simulink model "DCmotor_OL_Ctrl"  (R2022b)
settings: Solver=ode4  StartTime=0.0  StopTime=inf  FixedStep=0.001  RelTol=1e-3  EnableMultiTasking=on
libraries: arduinolib x5, arduinosensorlib x2
settings Model: ExtModeTrigDuration=2  Creator=user  LastModifiedBy=user
settings DataIOCC: ReturnWorkspaceOutputs=off
settings OptimizationCC: EnhancedBackFolding=on  PassReuseOutputArgsAs=Individual arguments  ZeroExternalMemoryAtStartup=off  ZeroInternalMemoryAtStartup=off  MaxStackSize=64  OptimizeBlockOrder=speed  DifferentSizesBufferReuse=on  OptimizationCustomize=off  EfficientTunableParamExpr=on
settings DebuggingCC: ParameterTunabilityLossMsg=error  UnconnectedInputMsg=warning  UnconnectedOutputMsg=warning  UnconnectedLineMsg=warning
settings HardwareCC: ProdBitPerInt=16  ProdBitPerPointer=16  ProdBitPerSizeT=16  ProdBitPerPtrDiffT=16  ProdLargestAtomicFloat=None  ProdWordSize=8  ProdHWDeviceType=Atmel->AVR
settings ModelReferenceCC: EnableRefExpFcnMdlSchedulingChecks=on
settings SFSimCC: MATLABDynamicMemAlloc=off
settings RTWCC: Description=Embedded Coder  SystemTargetFile=ert.tlc  HardwareBoard=Arduino Mega 2560  TLCOptions=-aInlineSetEventsForThisBaseRateFcn=TLC_FALSE -aSuppressMultiTaskScheduler=TLC_FALSE -aRateBasedStepFcn=1  TemplateMakefile=ert_default_tmf  Toolchain=Arduino AVR  BuildConfiguration=Faster Runs  DLArmComputeVersion=19.05
settings CodeAppCC: ForceParamTrailComments=on  IgnoreCustomStorageClasses=off  OperatorAnnotations=on  SimulinkDataObjDesc=on  SFDataObjDesc=on  InsertBlockDesc=on
settings ERTTargetCC: SupportContinuousTime=on  SupportVariableSizeSignals=on  ExtModeTransport=3  ExtModeStaticAlloc=on  ExtModeStaticAllocSize=2048  ExtModeMexFile=ext_xcp  ExtModeIntrfLevel=Level2 - Open

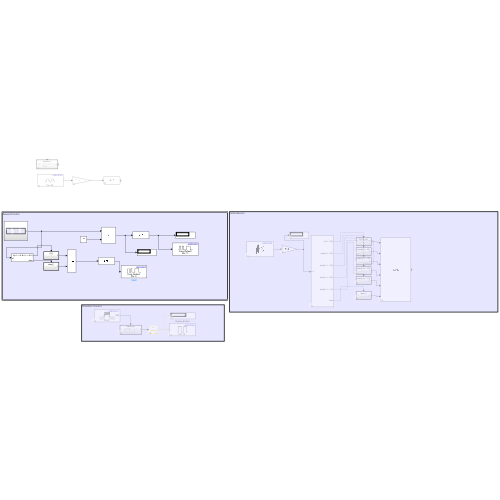
[thumbnail: Simulink's stored preview of the top-level diagram]
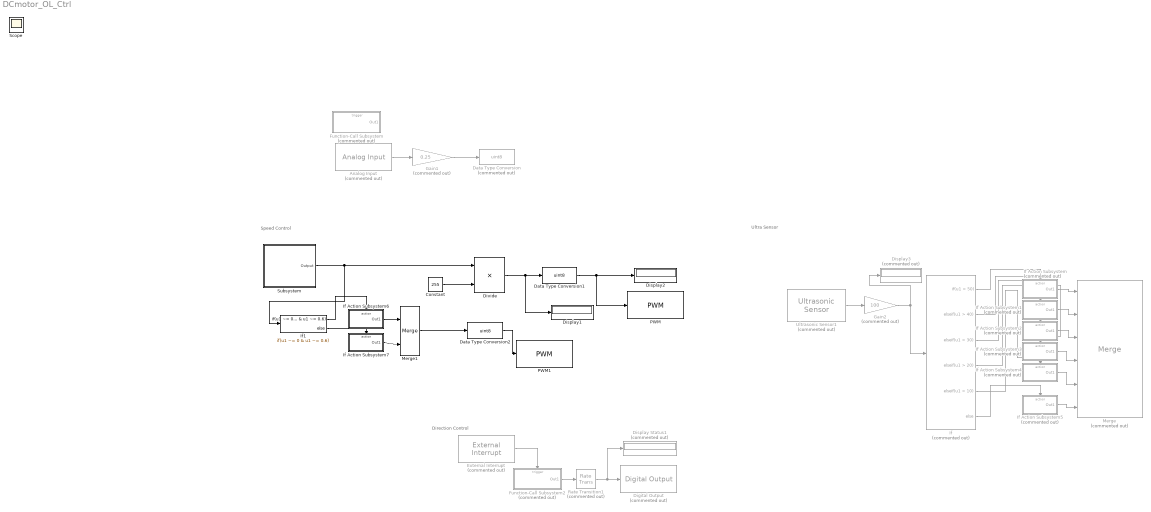
== system DCmotor_OL_Ctrl ==
  note: Speed Control
  note: Ultra Sensor
  note: Direction Control
  Analog Input : arduinolib/Analog Input  Commented=on  pinNumber=0  ReadResultsOnly=off  ConversionTriggerSource=Software  ExternalTriggerType=uint32( 0 )  OutputDataType=uint16  EnableConversionCompleteNotify=off  EnableOuputStatus=off  SampleTime=-1  blockPlatform=arduino
  Constant : Constant  Value=255
  Data Type Conversion : DataTypeConversion  Commented=on  OutDataTypeStr=uint8  SaturateOnIntegerOverflow=off  RndMeth=Floor
  Data Type Conversion1 : DataTypeConversion  OutDataTypeStr=uint8  SaturateOnIntegerOverflow=off  RndMeth=Floor
  Data Type Conversion2 : DataTypeConversion  OutDataTypeStr=uint8  SaturateOnIntegerOverflow=off  RndMeth=Floor
  Digital Output : arduinolib/Digital Output  Commented=on  pinNumber=13  Direction=output  blockPlatform=arduino
  Display Status1 : Display  Commented=on
  Display1 : Display
  Display2 : Display
  Display3 : Display  Commented=on
  Divide : Product  Inputs=**
  External Interrupt : arduinolib/External Interrupt  Commented=on  Pin=2  PullUp=off  Mode=FALLING  InterruptSimulationInput=off
  Function-Call Subsystem : Subsystem  Commented=on  TreatAsAtomicUnit=on
  Function-Call Subsystem2 : Subsystem  Commented=on  TreatAsAtomicUnit=on
  Gain1 : Gain  Commented=on  Gain=0.25
  Gain2 : Gain  Commented=on  Gain=100
  If : If  Commented=on  IfExpression=u1 > 50  ElseIfExpressions=u1 > 40, u1 > 30, u1 > 20, u1 > 10
  If Action Subsystem : Subsystem  Commented=on  TreatAsAtomicUnit=on
  If Action Subsystem1 : Subsystem  Commented=on  TreatAsAtomicUnit=on
  If Action Subsystem2 : Subsystem  Commented=on  TreatAsAtomicUnit=on
  If Action Subsystem3 : Subsystem  Commented=on  TreatAsAtomicUnit=on
  If Action Subsystem4 : Subsystem  Commented=on  TreatAsAtomicUnit=on
  If Action Subsystem5 : Subsystem  Commented=on  TreatAsAtomicUnit=on
  If Action Subsystem6 : Subsystem  TreatAsAtomicUnit=on
  If Action Subsystem7 : Subsystem  TreatAsAtomicUnit=on
  If1 : If  IfExpression=u1 ~= 0 & u1 ~= 0.6
  Merge : Merge  Commented=on  Inputs=6
  Merge1 : Merge  InitialOutput=[0]
  PWM : arduinolib/PWM  pinNumber=11  frequencyType=Default  desiredFrequency=490.2  achievableFrequency=490.2
  PWM1 : arduinolib/PWM  pinNumber=5  frequencyType=Default  desiredFrequency=490.2  achievableFrequency=490.2
  Rate Transition1 : RateTransition  Commented=on  Deterministic=off
  Subsystem : Subsystem
  Ultrasonic Sensor1 : arduinosensorlib/Ultrasonic Sensor  Commented=on  NumSignalPins=2  TrigPin=50  EchoPin=51  SignalPin=3  SampleTime_=0.1  blockPlatform=ARDUINO
  Scope : Scope
  wires:
  Analog Input/1 -> Gain1/1
  Gain1/1 -> Data Type Conversion/1
  Constant/1 -> Divide/2
  Data Type Conversion1/1 -> PWM/1, Display2/1
  Gain2/1 -> Display3/1, If/1
  Ultrasonic Sensor1/1 -> Gain2/1
  If/2 -> If Action Subsystem1/Action
  If/1 -> If Action Subsystem/Action
  If/3 -> If Action Subsystem2/Action
  If/4 -> If Action Subsystem3/Action
  If/5 -> If Action Subsystem4/Action
  If/6 -> If Action Subsystem5/Action
  If Action Subsystem/1(Out1) -> Merge/1
  If Action Subsystem1/1(Out1) -> Merge/2
  If Action Subsystem2/1(Out1) -> Merge/3
  If Action Subsystem3/1(Out1) -> Merge/4
  If Action Subsystem4/1(Out1) -> Merge/5
  If Action Subsystem5/1(Out1) -> Merge/6
  Divide/1 -> Display1/1, Data Type Conversion1/1
  Function-Call Subsystem2/1(Out1) -> Rate Transition1/1
  Rate Transition1/1 -> Display Status1/1, Digital Output/1
  External Interrupt/1 -> Function-Call Subsystem2/Trigger
  Subsystem/1(Output) -> Divide/1, If1/1
  Data Type Conversion2/1 -> PWM1/1
  If Action Subsystem6/1(Out1) -> Merge1/1
  If Action Subsystem7/1(Out1) -> Merge1/2
  If1/1 -> If Action Subsystem6/Action
  If1/2 -> If Action Subsystem7/Action
  Merge1/1 -> Data Type Conversion2/1

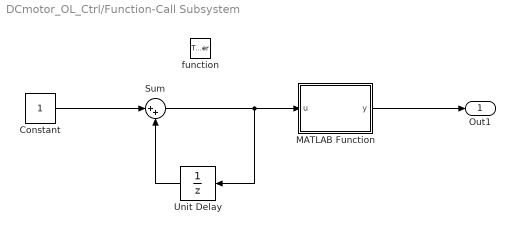
== system DCmotor_OL_Ctrl/Function-Call Subsystem ==
  function : TriggerPort  TriggerType=function-call  VariantControl=(inherit)
  Constant : Constant
  MATLAB Function : MATLAB Function  TreatAsAtomicUnit=on
  Sum : Sum  Inputs=|++
  Unit Delay : UnitDelay  SampleTime=-1  HasFrameUpgradeWarning=on
  Out1 : Outport
  wires:
  Constant/1 -> Sum/1
  Unit Delay/1 -> Sum/2
  Sum/1 -> Unit Delay/1, MATLAB Function/1(u)
  MATLAB Function/1(y) -> Out1/1

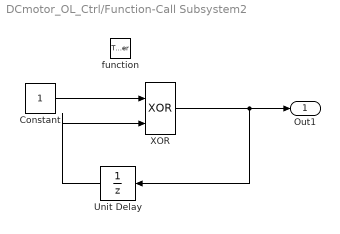
== system DCmotor_OL_Ctrl/Function-Call Subsystem2 ==
  function : TriggerPort  TriggerType=function-call  VariantControl=(inherit)
  Constant : Constant
  Unit Delay : UnitDelay  SampleTime=-1  HasFrameUpgradeWarning=on
  XOR : Logic  Operator=XOR  IconShape=distinctive  AllPortsSameDT=off  OutDataTypeStr=boolean
  Out1 : Outport
  wires:
  Constant/1 -> XOR/1
  Unit Delay/1 -> XOR/2
  XOR/1 -> Unit Delay/1, Out1/1

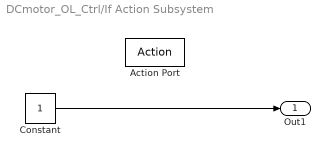
== system DCmotor_OL_Ctrl/If Action Subsystem ==
  Action Port : ActionPort  ActionPortLabel=if(u1 > 50)
  Constant : Constant
  Out1 : Outport
  wires:
  Constant/1 -> Out1/1

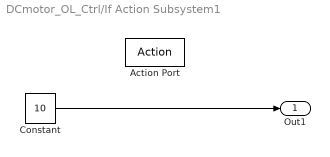
== system DCmotor_OL_Ctrl/If Action Subsystem1 ==
  Action Port : ActionPort  ActionPortLabel=elseif(u1 > 40)
  Constant : Constant  Value=10
  Out1 : Outport
  wires:
  Constant/1 -> Out1/1

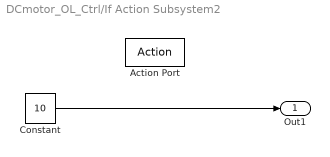
== system DCmotor_OL_Ctrl/If Action Subsystem2 ==
  Action Port : ActionPort  ActionPortLabel=elseif( u1 > 30)
  Constant : Constant  Value=10
  Out1 : Outport
  wires:
  Constant/1 -> Out1/1

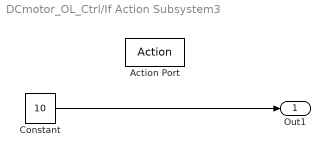
== system DCmotor_OL_Ctrl/If Action Subsystem3 ==
  Action Port : ActionPort  ActionPortLabel=elseif( u1 > 20)
  Constant : Constant  Value=10
  Out1 : Outport
  wires:
  Constant/1 -> Out1/1

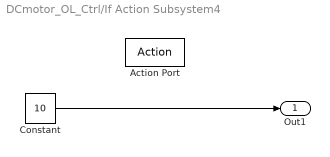
== system DCmotor_OL_Ctrl/If Action Subsystem4 ==
  Action Port : ActionPort  ActionPortLabel=elseif( u1 > 10)
  Constant : Constant  Value=10
  Out1 : Outport
  wires:
  Constant/1 -> Out1/1

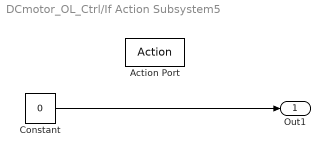
== system DCmotor_OL_Ctrl/If Action Subsystem5 ==
  Action Port : ActionPort  ActionPortLabel=else
  Constant : Constant  Value=0
  Out1 : Outport
  wires:
  Constant/1 -> Out1/1

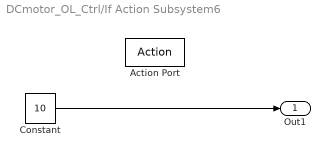
== system DCmotor_OL_Ctrl/If Action Subsystem6 ==
  Action Port : ActionPort  ActionPortLabel=if(u1 ~= 0 & u1 ~= 0.6)
  Constant : Constant  Value=10
  Out1 : Outport
  wires:
  Constant/1 -> Out1/1

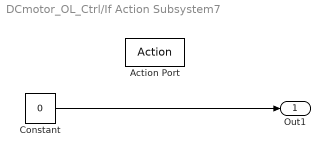
== system DCmotor_OL_Ctrl/If Action Subsystem7 ==
  Action Port : ActionPort  ActionPortLabel=else
  Constant : Constant  Value=0
  Out1 : Outport
  wires:
  Constant/1 -> Out1/1

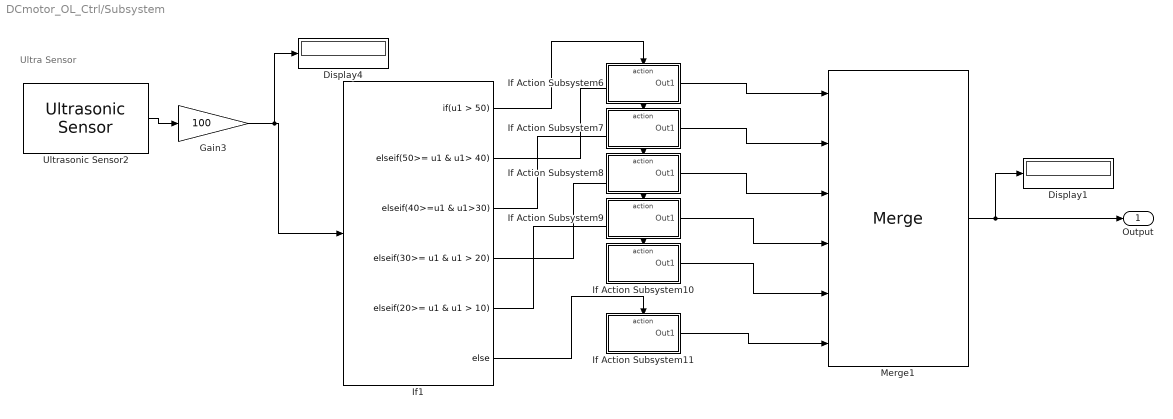
== system DCmotor_OL_Ctrl/Subsystem ==
  note: Ultra Sensor
  Display1 : Display
  Display4 : Display
  Gain3 : Gain  Gain=100
  If Action Subsystem10 : Subsystem  TreatAsAtomicUnit=on
  If Action Subsystem11 : Subsystem  TreatAsAtomicUnit=on
  If Action Subsystem6 : Subsystem  TreatAsAtomicUnit=on
  If Action Subsystem7 : Subsystem  TreatAsAtomicUnit=on
  If Action Subsystem8 : Subsystem  TreatAsAtomicUnit=on
  If Action Subsystem9 : Subsystem  TreatAsAtomicUnit=on
  If1 : If  IfExpression=u1 > 50  ElseIfExpressions=50>= u1 & u1> 40, 40>=u1 & u1>30, 30>= u1 & u1 > 20, 20>= u1 & u1 > 10
  Merge1 : Merge  Inputs=6
  Ultrasonic Sensor2 : arduinosensorlib/Ultrasonic Sensor  NumSignalPins=2  TrigPin=50  EchoPin=51  SignalPin=3  SampleTime_=0.1  blockPlatform=ARDUINO
  Output : Outport
  wires:
  Gain3/1 -> If1/1, Display4/1
  Ultrasonic Sensor2/1 -> Gain3/1
  If Action Subsystem9/1(Out1) -> Merge1/4
  If Action Subsystem11/1(Out1) -> Merge1/6
  If Action Subsystem8/1(Out1) -> Merge1/3
  If Action Subsystem7/1(Out1) -> Merge1/2
  If Action Subsystem6/1(Out1) -> Merge1/1
  If Action Subsystem10/1(Out1) -> Merge1/5
  If1/1 -> If Action Subsystem6/Action
  If1/2 -> If Action Subsystem7/Action
  If1/3 -> If Action Subsystem8/Action
  If1/4 -> If Action Subsystem9/Action
  If1/5 -> If Action Subsystem10/Action
  If1/6 -> If Action Subsystem11/Action
  Merge1/1 -> Display1/1, Output/1

== system DCmotor_OL_Ctrl/Subsystem/If Action Subsystem10 ==
  Action Port : ActionPort  ActionPortLabel=elseif( 20>= u1 & u1 > 10)
  Constant : Constant  Value=0.2
  Out1 : Outport
  wires:
  Constant/1 -> Out1/1

== system DCmotor_OL_Ctrl/Subsystem/If Action Subsystem11 ==
  Action Port : ActionPort  ActionPortLabel=else
  Constant : Constant  Value=0
  Out1 : Outport
  wires:
  Constant/1 -> Out1/1

== system DCmotor_OL_Ctrl/Subsystem/If Action Subsystem6 ==
  Action Port : ActionPort  ActionPortLabel=if(u1 > 50)
  Constant : Constant  Value=0.6
  Out1 : Outport
  wires:
  Constant/1 -> Out1/1

== system DCmotor_OL_Ctrl/Subsystem/If Action Subsystem7 ==
  Action Port : ActionPort  ActionPortLabel=elseif(50>= u1 & u1> 40)
  Constant : Constant  Value=0.5
  Out1 : Outport
  wires:
  Constant/1 -> Out1/1

== system DCmotor_OL_Ctrl/Subsystem/If Action Subsystem8 ==
  Action Port : ActionPort  ActionPortLabel=elseif( 40>=u1 & u1>30)
  Constant : Constant  Value=0.4
  Out1 : Outport
  wires:
  Constant/1 -> Out1/1

== system DCmotor_OL_Ctrl/Subsystem/If Action Subsystem9 ==
  Action Port : ActionPort  ActionPortLabel=elseif( 30>= u1 & u1 > 20)
  Constant : Constant  Value=0.3
  Out1 : Outport
  wires:
  Constant/1 -> Out1/1

== matlab function DCmotor_OL_Ctrl/Function-Call Subsystem/MATLAB Function ==
  data: u input; y output
function y = fcn(u)
 rem = mod(u,2);
 if rem == 0
     y=0;
 else
     y=1;
 end

 if u > 100
     u = 1;
 end
